simulink model "closedloop_statefeedback_estimator"  (R2015a)
settings: Solver=ode45  StartTime=0.0  StopTime=20  FixedStep=1e-3  MaxStep=1e-2  RelTol=1e-3
values from neighbouring files (symbols this model uses):
  A = [-2*xi*wn -wn^2 ... (first row only)    [script.m]
  B = [1 ... (first row only)    [script.m]
  C = [0 1/I]    [script.m]
  K1 = place(A,B,p)    [script.m]
  L = acker(A',C',p_obsv)'    [script.m]
  N1 = Nu+K1*Nx    [script.m]
libraries: simulink_extras x1
settings Model: Creator=henrik  LastModifiedBy=hg35a
settings DataIOCC: SignalLoggingSaveFormat=ModelDataLogs  SignalLoggingName=sigsOut
settings OptimizationCC: ExpressionDepthLimit=2147483647  InitFltsAndDblsToZero=on
settings DebuggingCC: SaveWithParameterizedLinksMsg=none  UnderspecifiedInitializationDetection=Classic  MergeDetectMultiDrivingBlocksExec=none  SignalResolutionControl=TryResolveAllWithWarning  MultiTaskDSMMsg=warning  MultiTaskCondExecSysMsg=none  FcnCallInpInsideContextMsg=UseLocalSettings  StateNameClashWarn=warning
settings HardwareCC: TargetUnknown=on
settings GRTTargetCC: TargetFcnLib=ansi_tfl_tmw.mat  ModelReferenceCompliant=off  CombineOutputUpdateFcns=off  MatFileLogging=off  GRTInterface=on

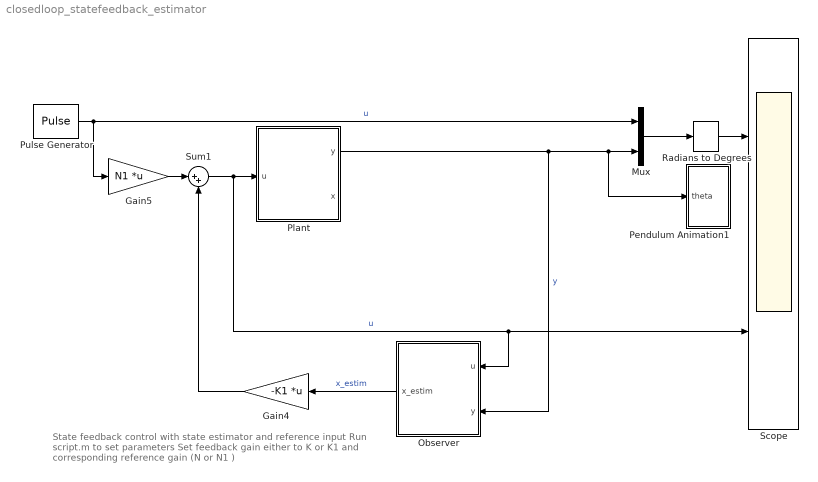
== system closedloop_statefeedback_estimator ==
  note: State feedback control with state estimator and reference input
      | Run script.m to set parameters
      | Set feedback gain either to K or K1
      | and corresponding reference gain (N or N1 )
  Gain4 : Gain  Gain=-K1  Multiplication=Matrix(K*u)  SaturateOnIntegerOverflow=on  OutDataTypeStr=Inherit: Same as input  ParamDataTypeStr=Inherit: Same as input
  Gain5 : Gain  Gain=N1  Multiplication=Matrix(K*u)  SaturateOnIntegerOverflow=on  OutDataTypeStr=Inherit: Same as input  ParamDataTypeStr=Inherit: Same as input
  Mux : Mux  Inputs=2
  Observer : Subsystem
  Pendulum Animation1 : Subsystem
  Plant : Subsystem
  Pulse Generator : DiscretePulseGenerator  PulseType=Time based  Amplitude=10*pi/180  Period=10  PulseWidth=50
      settings: AttributesFormatString=Amplitude=%<Amplitude>
  Radians to Degrees : simulink_extras/Transformations/Radians to Degrees
  Scope : Scope  NumInputPorts=2
      settings: YMin=-1~-17.5  YMax=11~17.5
  Sum1 : Sum  Inputs=|++
  wires:
  Pulse Generator/1 -> Mux/1, Gain5/1  "u"
  Mux/1 -> Radians to Degrees/1
  Sum1/1 -> Observer/1(u), Scope/2, Plant/1(u)  "u"
  Gain5/1 -> Sum1/1
  Radians to Degrees/1 -> Scope/1
  Gain4/1 -> Sum1/2
  Plant/1(y) -> Pendulum Animation1/1(theta), Mux/2, Observer/2(y)  "y"
  Observer/1(x_estim) -> Gain4/1  "x_estim"

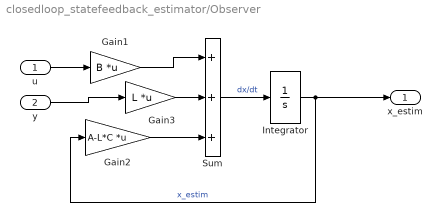
== system closedloop_statefeedback_estimator/Observer ==
  u : Inport
  y : Inport  Port=2
  Gain1 : Gain  Gain=B  Multiplication=Matrix(K*u)  SaturateOnIntegerOverflow=on  OutDataTypeStr=Inherit: Same as input  ParamDataTypeStr=Inherit: Same as input
  Gain2 : Gain  Gain=A-L*C  Multiplication=Matrix(K*u)  SaturateOnIntegerOverflow=on  OutDataTypeStr=Inherit: Same as input  ParamDataTypeStr=Inherit: Same as input
  Gain3 : Gain  Gain=L  Multiplication=Matrix(K*u)  SaturateOnIntegerOverflow=on  OutDataTypeStr=Inherit: Same as input  ParamDataTypeStr=Inherit: Same as input
  Integrator : Integrator
  Sum : Sum  Inputs=+++  SaturateOnIntegerOverflow=on  InputSameDT=on  OutDataTypeStr=Inherit: Same as first input
  x_estim : Outport
  wires:
  u/1 -> Gain1/1
  Sum/1 -> Integrator/1  "dx/dt"
  Integrator/1 -> Gain2/1, x_estim/1  "x_estim"
  Gain1/1 -> Sum/1
  Gain2/1 -> Sum/3
  y/1 -> Gain3/1
  Gain3/1 -> Sum/2

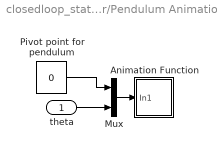
== system closedloop_statefeedback_estimator/Pendulum Animation1 ==
  theta : Inport
  Animation Function : Subsystem  mask(Animation Block){ts=0.01}
      mask prompts: ts "Sample time:"
      mask Display: plot([.1,.9],[.9,.9],[.5,.2],[.9,.25],[.475,.475,.525,.525,.475],[.875,.925,.925,.875,.875])
  Mux : Mux  Inputs=2
  Pivot point for pendulum : Constant  Value=0
  wires:
  theta/1 -> Mux/2
  Pivot point for pendulum/1 -> Mux/1
  Mux/1 -> Animation Function/1(In1)

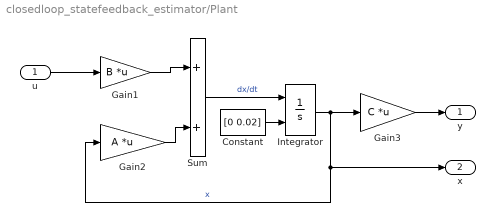
== system closedloop_statefeedback_estimator/Plant ==
  u : Inport
  Constant : Constant  Value=[0 0.02]
  Gain1 : Gain  Gain=B  Multiplication=Matrix(K*u)  SaturateOnIntegerOverflow=on  OutDataTypeStr=Inherit: Same as input  ParamDataTypeStr=Inherit: Same as input
  Gain2 : Gain  Gain=A  Multiplication=Matrix(K*u)  SaturateOnIntegerOverflow=on  OutDataTypeStr=Inherit: Same as input  ParamDataTypeStr=Inherit: Same as input
  Gain3 : Gain  Gain=C  Multiplication=Matrix(K*u)  SaturateOnIntegerOverflow=on  OutDataTypeStr=Inherit: Same as input  ParamDataTypeStr=Inherit: Same as input
  Integrator : Integrator  InitialConditionSource=external
  Sum : Sum  SaturateOnIntegerOverflow=on  InputSameDT=on  OutDataTypeStr=Inherit: Same as first input
  y : Outport
  x : Outport  Port=2
  wires:
  Gain1/1 -> Sum/1
  Constant/1 -> Integrator/2
  Gain2/1 -> Sum/2
  Integrator/1 -> Gain3/1, Gain2/1, x/1  "x"
  Sum/1 -> Integrator/1  "dx/dt"
  Gain3/1 -> y/1
  u/1 -> Gain1/1

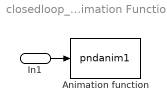
== system closedloop_statefeedback_estimator/Pendulum Animation1/Animation Function ==
  In1 : Inport
  Animation function : S-Function  FunctionName=pndanim1  Parameters=ts
      settings: DeleteFcn=if ~isempty(findobj('type','figure','name','simppend Animation'));close('simppend Animation'); end;
  wires:
  In1/1 -> Animation function/1
